simulink model "NDI_reference_shaping_example"  (R2023a)
settings: Solver=FixedStepAuto  StartTime=0.0  StopTime=25  FixedStep=0.001  RelTol=1e-3
undefined symbols (not defined in the file or in its folder): frameRate_hz
settings Model: Creator=abhandari1  LastModifiedBy=abhandari1

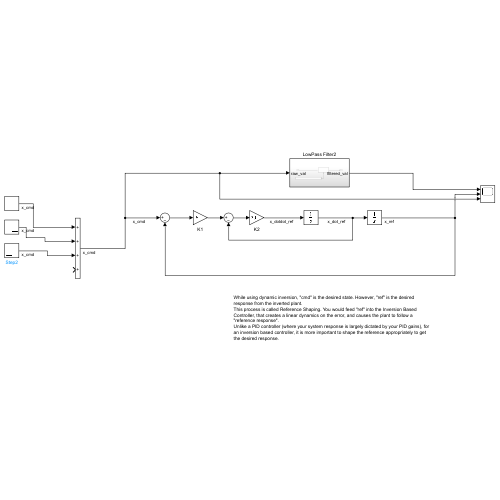
[thumbnail: Simulink's stored preview of the top-level diagram]
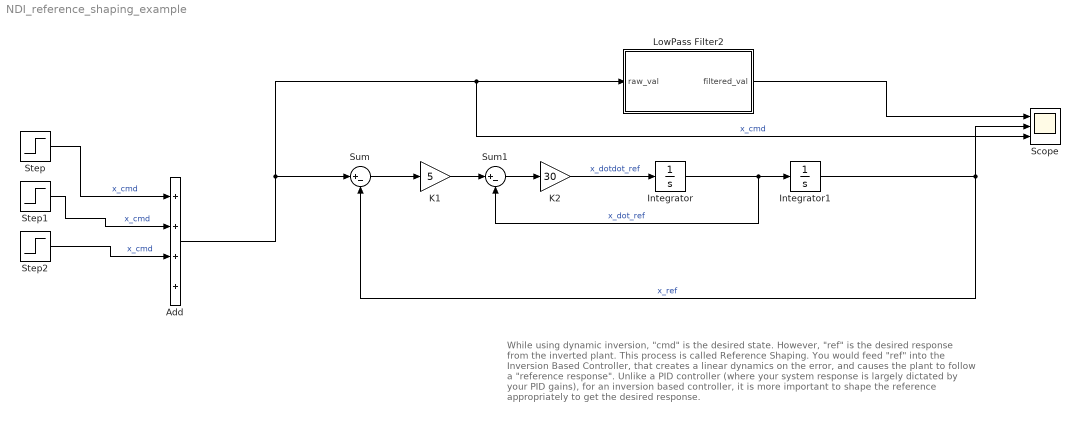
== system NDI_reference_shaping_example ==
  note: While using dynamic inversion, "cmd" is the desired state. However, "ref" is the desired response from the inverted plant.
      | This process is called Reference Shaping. You would feed "ref" into the Inversion Based Controller, that creates a linear dynamics on the error, and causes the plant to follow a "reference response".
      | Unlike a PID controller (where your system response is largely dictated by your PID gains), for an inversion based controller, it is more important to shape the reference appropriately to get the desired response.
  Add : Sum  Inputs=++++
  Integrator : Integrator
  Integrator1 : Integrator
  K1 : Gain  Gain=5
  K2 : Gain  Gain=30
  LowPass Filter2 : Subsystem
      settings: PortSchema="{\"entries\":[{\"content\":{\"sides\":[{\"content\":{\"connectorIds\":[\"Out1\"]},\"type\":\"ConnectorPlacement.EquallySpacedRectSide\",\"uuid\":\"91cc3e13-2b14-472d-8884-d1975898cd34\"},{\"content\":{\"connectorIds\":[\"In1\"],\"side\":\"RIGHT\"},\"type\":\"ConnectorPlacement.EquallySpacedRectSide\",\"uuid\":\"ce6b3021-6e32-4737-8c8e-25014706d3dd\"},{\"content\":{\"side\":\"TOP\"},\"type\":\"ConnectorPlacement.EquallySpacedRectSide\",\"uuid\":\"ad734f0b-b067-43e6-a641-0e0955250a7f\"},{\"content\":{\"side\":\"BOTTOM\"},\"type\":\"ConnectorPlacement.EquallySpacedRectSide\",\"uuid\":\"618c62c8-d4e2-4678-9fe1-905e2f147d5d\"}]},\"type\":\"ConnectorPlacement.EquallySpacedConnector\",\"uuid\":\"c0097053-d36a-473a-84fb-0616f69f4bc5\"}],\"packageUris\":[\"http://schema.mathworks.com/mf0/Connector/R2020b\"],\"version\":\"1.0\"}"
  Scope : Scope  NumInputPorts=3
  Step : Step  SampleTime=0
  Step1 : Step  Time=9  Before=1  After=-1  SampleTime=0
  Step2 : Step  Time=17  Before=-1  After=0  SampleTime=0
  Sum : Sum  Inputs=|+-
  Sum1 : Sum  Inputs=|+-
  wires:
  Step/1 -> Add/1  "x_cmd"
  Step1/1 -> Add/2  "x_cmd"
  Step2/1 -> Add/3  "x_cmd"
  LowPass Filter2/1(filtered_val) -> Scope/1
  Integrator1/1 -> Sum/2, Scope/2  "x_ref"
  Sum1/1 -> K2/1
  Add/1 -> Sum/1, Scope/3, LowPass Filter2/1(raw_val)  "x_cmd"
  Integrator/1 -> Sum1/2, Integrator1/1  "x_dot_ref"
  Sum/1 -> K1/1
  K2/1 -> Integrator/1  "x_dotdot_ref"
  K1/1 -> Sum1/1

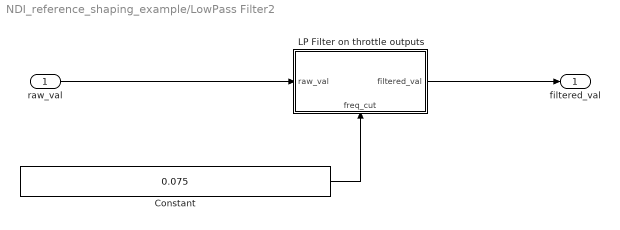
== system NDI_reference_shaping_example/LowPass Filter2 ==
  raw_val : Inport
  Constant : Constant  Value=0.075
  LP Filter on throttle outputs : Subsystem
      settings: PortSchema="{\"entries\":[{\"content\":{\"sides\":[{\"content\":{\"connectorIds\":[\"In1\"]},\"type\":\"ConnectorPlacement.EquallySpacedRectSide\",\"uuid\":\"20236834-aeb3-4c5b-bb2e-f84447e752b5\"},{\"content\":{\"connectorIds\":[\"Out1\"],\"side\":\"RIGHT\"},\"type\":\"ConnectorPlacement.EquallySpacedRectSide\",\"uuid\":\"d668f9a1-a3df-4207-8bf1-99fb838e59b2\"},{\"content\":{\"connectorIds\":[],\"side\":\"TOP\"},\"type\":\"ConnectorPlacement.EquallySpacedRectSide\",\"uuid\":\"66cceb06-f4bc-4278-b965-2427292e46df\"},{\"content\":{\"connectorIds\":[\"In2\"],\"side\":\"BOTTOM\"},\"type\":\"ConnectorPlacement.EquallySpacedRectSide\",\"uuid\":\"8fdaac6a-cb03-4bd4-87bb-7bafd10bc297\"}]},\"type\":\"ConnectorPlacement.EquallySpacedConnector\",\"uuid\":\"3dc29a9a-e794-478d-b7df-452e6c2d3f66\"}],\"packageUris\":[\"http://schema.mathworks.com/mf0/Connector/R2020b\"],\"version\":\"1.0\"}"
  filtered_val : Outport
  wires:
  raw_val/1 -> LP Filter on throttle outputs/1(raw_val)
  Constant/1 -> LP Filter on throttle outputs/2(freq_cut)
  LP Filter on throttle outputs/1(filtered_val) -> filtered_val/1

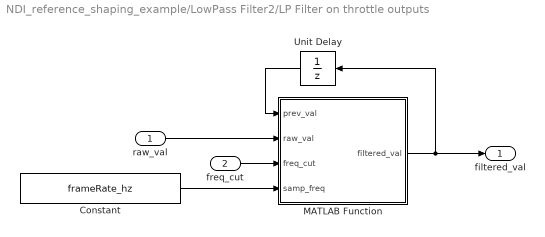
== system NDI_reference_shaping_example/LowPass Filter2/LP Filter on throttle outputs ==
  raw_val : Inport
  freq_cut : Inport  Port=2
  Constant : Constant  Value=frameRate_hz  OutDataTypeStr=single
  MATLAB Function : MATLAB Function  TreatAsAtomicUnit=on
  Unit Delay : UnitDelay  SampleTime=-1  HasFrameUpgradeWarning=on
  filtered_val : Outport
  wires:
  freq_cut/1 -> MATLAB Function/3(freq_cut)
  MATLAB Function/1(filtered_val) -> Unit Delay/1, filtered_val/1
  Unit Delay/1 -> MATLAB Function/1(prev_val)
  raw_val/1 -> MATLAB Function/2(raw_val)
  Constant/1 -> MATLAB Function/4(samp_freq)

== matlab function NDI_reference_shaping_example/LowPass Filter2/LP Filter on throttle outputs/MATLAB Function ==
  data: prev_val input single; raw_val input; filtered_val output; freq_cut input; samp_freq input
function filtered_val = IIR_filt( prev_val,raw_val, freq_cut, samp_freq)
    fc = freq_cut/samp_freq;
    b = 2 - cos(2 * pi * fc) - sqrt((2 - cos(2 * pi * fc))^2 - 1);
    a = 1 - b;
    filtered_val = a * raw_val + b * prev_val;
